simulink model "Transient_Response"  (R2018a)
settings: Solver=VariableStepAuto  StartTime=0.0  StopTime=10.0  RelTol=1e-3
settings Model: Creator=vardh  LastModifiedBy=vardh

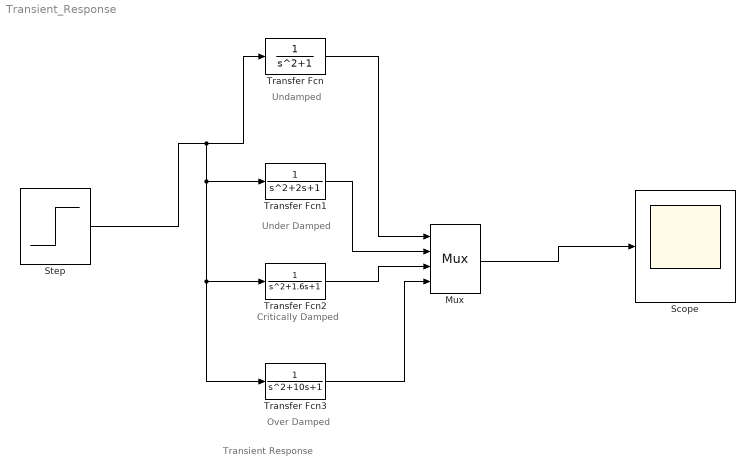
== system Transient_Response ==
  note: Transient Response
  note: Over Damped
  note: Critically Damped
  note: Under Damped
  note: Undamped
  Mux : Mux
  Scope : Scope
  Step : Step  SampleTime=0
  Transfer Fcn : TransferFcn  Numerator=[ 1]  Denominator="[1  0 1]"
  Transfer Fcn1 : TransferFcn
  Transfer Fcn2 : TransferFcn  Denominator=[1 1.6 1]
  Transfer Fcn3 : TransferFcn  Denominator=[1 10 1]
  wires:
  Step/1 -> Transfer Fcn3/1, Transfer Fcn2/1, Transfer Fcn1/1, Transfer Fcn/1
  Transfer Fcn/1 -> Mux/1
  Transfer Fcn1/1 -> Mux/2
  Transfer Fcn2/1 -> Mux/3
  Transfer Fcn3/1 -> Mux/4
  Mux/1 -> Scope/1
